simulink model "RL_TF_SS_1"  (R2023b)
settings: Solver=VariableStepAuto  StartTime=0.0  StopTime=0.002  MaxStep=1e-4  RelTol=1e-4  EnableMultiTasking=on
values from neighbouring files (symbols this model uses):
  Ts = 1e-6    (= 1e-06)    [RL_AC_2.m]
libraries: rllib x1
settings Model: SimulationMode=accelerator  Creator=The MathWorks, Inc.  LastModifiedBy=User
settings SolverCC: AlgebraicLoopSolver=TrustRegion  SolverResetMethod=Robust
settings OptimizationCC: LifeSpan=inf
settings DebuggingCC: ReadBeforeWriteMsg=DisableAll  WriteAfterWriteMsg=DisableAll  WriteAfterReadMsg=DisableAll  MultiTaskDSMMsg=none  UnconnectedInputMsg=warning  UnconnectedOutputMsg=warning  UnconnectedLineMsg=warning  SFUnexpectedBacktrackingDiag=warning  SFNoUnconditionalDefaultTransitionDiag=warning  SFExecutionAtInitializationDiag=none  ArithmeticOperatorsInVariantConditions=warning
settings ModelReferenceCC: UpdateModelReferenceTargets=IfOutOfDate  EnableRefExpFcnMdlSchedulingChecks=on
settings SFSimCC: SFSimEcho=off  SimUseLocalCustomCode=off  CustomCodeUndefinedFunction=UseInterfaceOnly
settings RTWCC: RTWUseLocalCustomCode=off
settings CodeAppCC: StateflowObjectComments=on
settings GRTTargetCC: TargetLangStandard=C89/C90 (ANSI)
settings ConfigComp: CovMetricSettings=dw  CovSaveCumulativeToWorkspaceVar=on  CovSaveSingleToWorkspaceVar=on  CovExternalEMLEnable=off
settings SimscapeCC: SimscapeNormalizeSystem=off  SimscapeNominalValues={1, 'bar'; 1, 'cm^3/s'; 1, 'bar*kg/s'; 1, 'kJ/kg'; 1, 'kW'; }

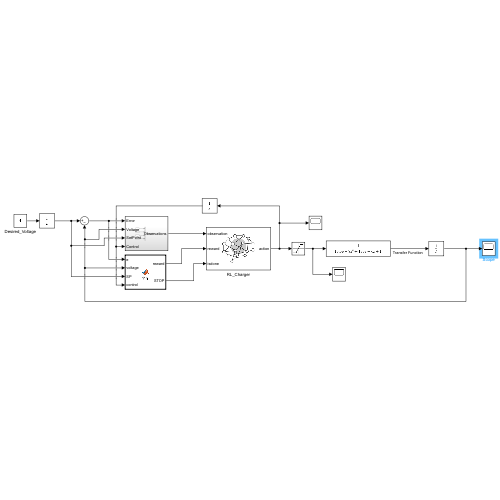
[thumbnail: Simulink's stored preview of the top-level diagram]
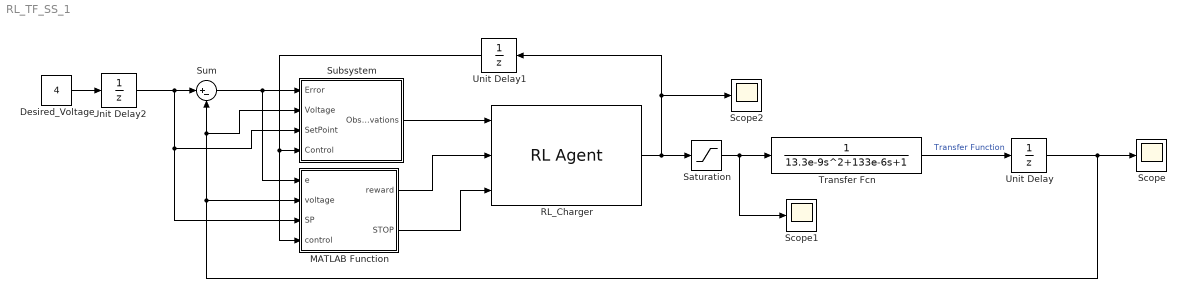
== system RL_TF_SS_1 ==
  Desired_Voltage : Constant  Value=4
  MATLAB Function : MATLAB Function  TreatAsAtomicUnit=on
  RL_Charger : rllib/RL Agent  Agent=agent  ExternalActionAsInput=off  ProvideLastAction=off  ProvideCumRwd=off  TreatAsDirectFeedthrough=on  UseStrictObservationDataTypes=off
  Saturation : Saturate  UpperLimit=10  LowerLimit=0
  Scope : Scope
  Scope1 : Scope
  Scope2 : Scope
  Subsystem : Subsystem
  Sum : Sum  Inputs=|+-
  Transfer Fcn : TransferFcn  Denominator=[13.3e-9 133e-6 1]
  Unit Delay : UnitDelay  SampleTime=Ts  HasFrameUpgradeWarning=on
  Unit Delay1 : UnitDelay  SampleTime=Ts  HasFrameUpgradeWarning=on
  Unit Delay2 : UnitDelay  SampleTime=Ts  HasFrameUpgradeWarning=on
  wires:
  Subsystem/1(Observations) -> RL_Charger/1
  MATLAB Function/1(reward) -> RL_Charger/2
  MATLAB Function/2(STOP) -> RL_Charger/3
  Desired_Voltage/1 -> Unit Delay2/1
  Sum/1 -> MATLAB Function/1(e), Subsystem/1(Error)
  Transfer Fcn/1 -> Unit Delay/1  "Transfer Function"
  Unit Delay/1 -> Scope/1, Subsystem/2(Voltage), Sum/2, MATLAB Function/2(voltage)
  Unit Delay1/1 -> MATLAB Function/4(control), Subsystem/4(Control)
  Unit Delay2/1 -> MATLAB Function/3(SP), Subsystem/3(SetPoint), Sum/1
  Saturation/1 -> Scope1/1, Transfer Fcn/1
  RL_Charger/1 -> Saturation/1, Unit Delay1/1, Scope2/1

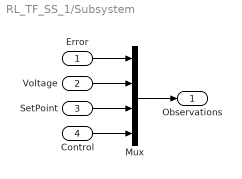
== system RL_TF_SS_1/Subsystem ==
  Error : Inport
  Voltage : Inport  Port=2
  SetPoint : Inport  Port=3
  Control : Inport  Port=4
  Mux : Mux
  Observations : Outport
  wires:
  Mux/1 -> Observations/1
  Error/1 -> Mux/1
  Voltage/1 -> Mux/2
  SetPoint/1 -> Mux/3
  Control/1 -> Mux/4

== matlab function RL_TF_SS_1/MATLAB Function ==
  data: e input; reward output; voltage input; STOP output; SP input; control input
% Función de recompensa
function [reward, STOP] = fcn(e, voltage, SP, control)
    % Función de recompensa ajustada
    ce1 = 200 * (abs(e) <= 0.5); % Recompensa alta para errores pequeños
    ce2 = -25 * (abs(e) > 0.5); % Penalización moderada para errores grandes
    cv = -10 * (voltage > 4); % Penalización moderada para corriente alta
    cc = 180 * (control == SP);
    % Calcular la recompensa total
    reward = ce1 + ce2 + cv + cc;

    % Condición de parada
    STOP = false; % Detener el episodio si el voltaje excede 24
end
